simulink model "network_motif_controller_linear_biological_optimisehill"  (R2022b)
settings: Solver=ode4  StartTime=0.0  StopTime=8000-0*5950  FixedStep=0.1  RelTol=1e-3
settings Model: Creator=u1473578  LastModifiedBy=u1473578
settings DebuggingCC: UnconnectedInputMsg=warning  UnconnectedOutputMsg=warning  UnconnectedLineMsg=warning
settings ModelReferenceCC: EnableRefExpFcnMdlSchedulingChecks=on
settings RTWCC: DLArmComputeVersion=19.05

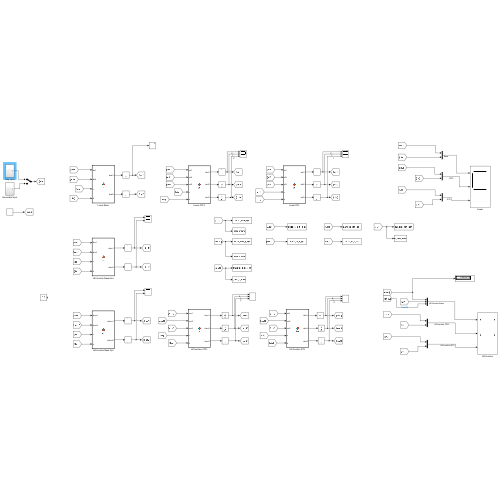
[thumbnail: Simulink's stored preview of the top-level diagram]
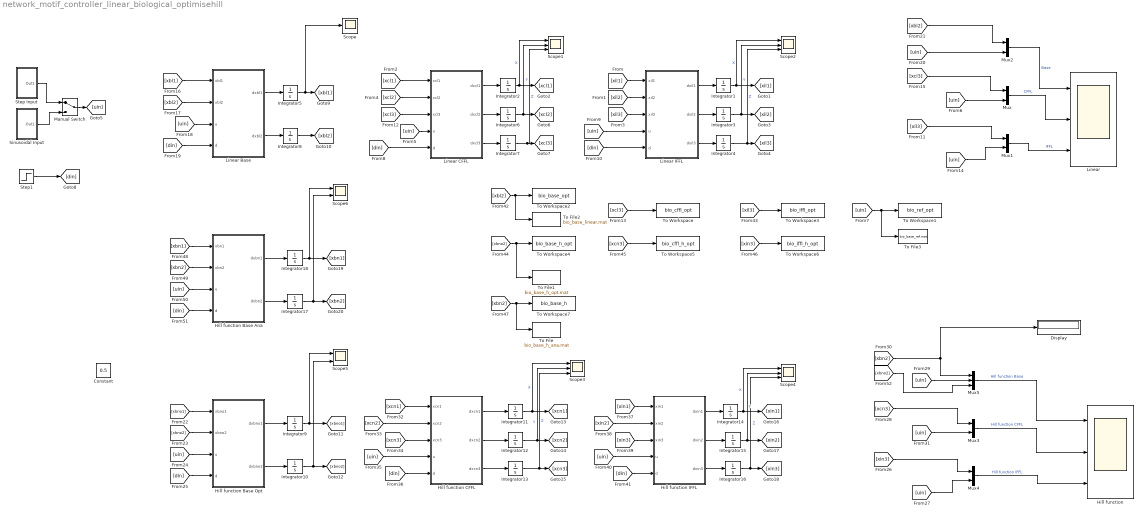
== system network_motif_controller_linear_biological_optimisehill ==
  Constant : Constant  Value=0.5
  Display : Display
  Hill function : Scope  NumInputPorts=3
  Hill function Base Ana : MATLAB Function  TreatAsAtomicUnit=on
  Hill function Base Opt : MATLAB Function  TreatAsAtomicUnit=on
  Hill function CFFL : MATLAB Function  TreatAsAtomicUnit=on
  Hill function IFFL : MATLAB Function  TreatAsAtomicUnit=on
  Integrator{1..18} (18 alike) : Integrator
  Linear : Scope  NumInputPorts=3
  Linear Base : MATLAB Function  TreatAsAtomicUnit=on
  Linear CFFL : MATLAB Function  TreatAsAtomicUnit=on
  Linear IFFL : MATLAB Function  TreatAsAtomicUnit=on
  Manual Switch : ManualSwitch
  Mux{,1..4} (5 alike) : Mux  Inputs=2
  Mux5 : Mux  Inputs=3
  Scope : Scope
  Scope{1..4} (4 alike) : Scope  NumInputPorts=3
  Scope5 : Scope  NumInputPorts=2
  Scope6 : Scope  NumInputPorts=2
  Sinusoidal Input : Subsystem
  Step Input : Subsystem
  Step1 : Step  Time=3000-0*1000  After=1*0.05*(-5e-4)  SampleTime=0
  To File : ToFile  Filename=bio_base_h_ana.mat  MatrixName=xbna2  SaveFormat=Timeseries
  To File1 : ToFile  Filename=bio_base_h_opt.mat  MatrixName=xbno2  SaveFormat=Timeseries
  To File2 : ToFile  Filename=bio_base_linear.mat  MatrixName=xbl2  SaveFormat=Timeseries
  To File3 : ToFile  Filename=bio_base_ref.mat  MatrixName=uref  SaveFormat=Timeseries
  To Workspace : ToWorkspace  VariableName=bio_cffl_opt  SaveFormat=Timeseries  SampleTime=-1
  To Workspace1 : ToWorkspace  VariableName=bio_ref_opt  SaveFormat=Timeseries  SampleTime=-1
  To Workspace2 : ToWorkspace  VariableName=bio_base_opt  SaveFormat=Timeseries  SampleTime=-1
  To Workspace3 : ToWorkspace  VariableName=bio_iffl_opt  SaveFormat=Timeseries  SampleTime=-1
  To Workspace4 : ToWorkspace  VariableName=bio_base_h_opt  SaveFormat=Timeseries  SampleTime=-1
  To Workspace5 : ToWorkspace  VariableName=bio_cffl_h_opt  SaveFormat=Timeseries  SampleTime=-1
  To Workspace6 : ToWorkspace  VariableName=bio_iffl_h_opt  SaveFormat=Timeseries  SampleTime=-1
  To Workspace7 : ToWorkspace  VariableName=bio_base_h  SaveFormat=Timeseries  SampleTime=-1
  wires:
  Integrator2/1 -> Scope1/1, [xcl1]  "X"
  Linear CFFL/3(dxcl3) -> Integrator7/1
  [xcl1] -> Linear CFFL/1(xcl1)
  Integrator7/1 -> Scope1/3, [xcl3]  "Z"
  [xcl2] -> Linear CFFL/2(xcl2)
  [xcl3] -> Linear CFFL/3(xcl3)
  Linear CFFL/2(dxcl2) -> Integrator6/1
  Integrator6/1 -> Scope1/2, [xcl2]  "Y"
  Linear CFFL/1(dxcl1) -> Integrator2/1
  Step Input/1(Out1) -> Manual Switch/1
  Sinusoidal Input/1(Out1) -> Manual Switch/2
  Linear IFFL/1(dxil1) -> Integrator1/1
  Linear IFFL/2(dxil2) -> Integrator3/1
  Linear IFFL/3(dxil3) -> Integrator4/1
  Integrator1/1 -> Scope2/1, [xil1]  "X"
  Integrator3/1 -> Scope2/2, [xil2]  "Y"
  Integrator4/1 -> Scope2/3, [xil3]  "Z"
  [xil1] -> Linear IFFL/1(xil1)
  [xil2] -> Linear IFFL/2(xil2)
  [xil3] -> Linear IFFL/3(xil3)
  Manual Switch/1 -> [uin]
  [uin] -> Linear CFFL/4(u)
  [uin] -> To File3/1, To Workspace1/1
  Step1/1 -> [din]
  [din] -> Linear CFFL/5(d)
  [uin] -> Linear IFFL/4(u)
  [din] -> Linear IFFL/5(d)
  [xcl3] -> To Workspace/1
  Mux/1 -> Linear/2  "CFFL"
  Mux1/1 -> Linear/3  "IFFL"
  [uin] -> Mux/2
  [xcl3] -> Mux/1
  [xil3] -> Mux1/1
  [uin] -> Mux1/2
  Linear Base/1(dxbl1) -> Integrator5/1
  Linear Base/2(dxbl2) -> Integrator8/1
  Integrator5/1 -> Scope/1, [xbl1]
  Integrator8/1 -> [xbl2]
  [xbl1] -> Linear Base/1(xbl1)
  [xbl2] -> Linear Base/2(xbl2)
  [uin] -> Linear Base/3(u)
  [din] -> Linear Base/4(d)
  Mux2/1 -> Linear/1  "Base"
  [xbl2] -> Mux2/1
  [uin] -> Mux2/2
  Hill function Base Opt/1(dxbno1) -> Integrator9/1
  Hill function Base Opt/2(dxbno2) -> Integrator10/1
  Integrator9/1 -> Scope5/1, [xbno1]
  Integrator10/1 -> Scope5/2, [xbno2]
  [xbno1] -> Hill function Base Opt/1(xbno1)
  [xbno2] -> Hill function Base Opt/2(xbno2)
  [din] -> Hill function Base Opt/4(d)
  [xbn2] -> Mux5/1, Display/1
  Mux5/1 -> Hill function/1  "Hill function Base"
  [uin] -> Mux4/2
  [xin3] -> Mux4/1
  [xcn3] -> Mux3/1
  [uin] -> Mux3/2
  Mux4/1 -> Hill function/3  "Hill function IFFL"
  Mux3/1 -> Hill function/2  "Hill function CFFL"
  Hill function CFFL/1(dxcn1) -> Integrator11/1
  Hill function CFFL/2(dxcn2) -> Integrator12/1
  Hill function CFFL/3(dxcn3) -> Integrator13/1
  [xcn1] -> Hill function CFFL/1(xcn1)
  [xcn2] -> Hill function CFFL/2(xcn2)
  [xcn3] -> Hill function CFFL/3(xcn3)
  [uin] -> Hill function CFFL/4(u)
  [din] -> Hill function CFFL/5(d)
  Integrator11/1 -> Scope3/1, [xcn1]  "X"
  Integrator12/1 -> Scope3/2, [xcn2]  "Y"
  Integrator13/1 -> Scope3/3, [xcn3]  "Z"
  Hill function IFFL/1(dxin1) -> Integrator14/1
  Hill function IFFL/2(dxin2) -> Integrator15/1
  Hill function IFFL/3(dxin3) -> Integrator16/1
  Integrator14/1 -> Scope4/1, [xin1]  "X"
  Integrator15/1 -> Scope4/2, [xin2]  "Y"
  Integrator16/1 -> Scope4/3, [xin3]  "Z"
  [xin1] -> Hill function IFFL/1(xin1)
  [xin2] -> Hill function IFFL/2(xin2)
  [xin3] -> Hill function IFFL/3(xin3)
  [uin] -> Hill function IFFL/4(u)
  [din] -> Hill function IFFL/5(d)
  [xbl2] -> To File2/1, To Workspace2/1
  [xil3] -> To Workspace3/1
  [uin] -> Hill function Base Opt/3(u)
  [xbno2] -> To File1/1, To Workspace4/1
  [xcn3] -> To Workspace5/1
  [xin3] -> To Workspace6/1
  [xbn2] -> To File/1, To Workspace7/1
  Hill function Base Ana/1(dxbn1) -> Integrator18/1
  [din] -> Hill function Base Ana/4(d)
  [xbn2] -> Hill function Base Ana/2(xbn2)
  Integrator17/1 -> Scope6/2, [xbn2]
  [uin] -> Hill function Base Ana/3(u)
  [xbn1] -> Hill function Base Ana/1(xbn1)
  Integrator18/1 -> Scope6/1, [xbn1]
  Hill function Base Ana/2(dxbn2) -> Integrator17/1
  [uin] -> Mux5/2
  [xbno2] -> Mux5/3

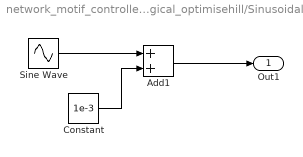
== system network_motif_controller_linear_biological_optimisehill/Sinusoidal Input ==
  Add1 : Sum
  Constant : Constant  Value=1e-3
  Sine Wave : Sin  Amplitude=1e-3  Frequency=10/6000  Phase=2800-150  SampleTime=0
  Out1 : Outport
  wires:
  Sine Wave/1 -> Add1/1
  Constant/1 -> Add1/2
  Add1/1 -> Out1/1

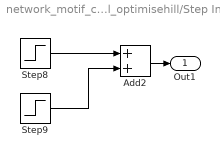
== system network_motif_controller_linear_biological_optimisehill/Step Input ==
  Add2 : Sum
  Step8 : Step  Time=0  After=0  SampleTime=0
  Step9 : Step  Time=1000  After=1e-3  SampleTime=0
  Out1 : Outport
  wires:
  Step9/1 -> Add2/2
  Step8/1 -> Add2/1
  Add2/1 -> Out1/1

== matlab function network_motif_controller_linear_biological_optimisehill/Linear IFFL ==
  data: xil1 input; xil2 input; xil3 input; u input; dxil1 output; dxil2 output; d input; dxil3 output
function [dxil1,dxil2,dxil3] = fcn(xil1,xil2,xil3,u,d)

% x1 = X
% x2 = Y
% x3 = Z

gamma = 1;
c = gamma;
% % per second
% delta_x = 0.001;
% delta_y = 0.004;
% delta_z = 0.004;

% per minutes
delta_x = 0.0005;
delta_y = 0.02;
delta_z = 0.02;

% % per hour
% delta_x = 0.0013;
% delta_y = 0.1;
% delta_z = 0.1;

alpha_y = 0.0005;
alpha_z1 = 0.0005;
alpha_z2 = 0.0005;



dxil1 = c*u - gamma*xil3 - delta_x*xil1;

dxil2 = alpha_y*xil1 - delta_y*xil2;

dxil3 = alpha_z1*xil1 - alpha_z2*xil2 - delta_z*xil3 + 1*d;

== matlab function network_motif_controller_linear_biological_optimisehill/Linear Base ==
  data: xbl1 input; xbl2 input; u input; dxbl1 output; dxbl2 output; d input
function [dxbl1,dxbl2] = fcn(xbl1,xbl2,u,d)

% x1 = X
% x2 = Z

gamma = 1;
c = gamma;

% % per second
% delta_x = 0.001;
% delta_y = 0.004;
% delta_z = 0.004;

% per minutes
delta_x = 0.0005;
delta_z = 0.02;

% % per hour
% delta_x = 0.0013;
% delta_y = 0.1;
% delta_z = 0.1;

alpha_z = 0.0005;


bs = 0*5e-3;

dxbl1 = c*u - gamma*xbl2 - delta_x*xbl1 + bs;

dxbl2 = alpha_z*xbl1 - delta_z*xbl2 + 1*d;

== matlab function network_motif_controller_linear_biological_optimisehill/Hill function Base Opt ==
  data: xbno1 input; xbno2 input; u input; dxbno1 output; dxbno2 output; d input
function [dxbno1,dxbno2] = fcn(xbno1,xbno2,u,d)

% x1 = X
% x2 = Z

gamma = 1;
c = gamma;
%% Derived Parameters through two-point matching (Inhibition Type 1)
% Kx = 0.002;
% Kz = 0.08;
% 
% % per minutes
% delta_x = 0.0005;
% delta_z = 0.02;
% 
% alpha_x = 2e-8;
% alpha_z = 1e-4;
% 
% bs = -5e-3;

%% Derived Parameters through two-point matching (Inhibition Type 2)
% Kx = 0.002; % analytic
Kx = 0.0022; % optimise
% Kz = 0.08; % analytic
Kz = 0.1896; % optimise

% per minutes
delta_x = 0.0005;
delta_z = 0.02;

% alpha_x = 0.005; % analytic
alpha_x = 0.0051; % optimise
% alpha_z = 1e-4; % analytic
alpha_z = 2e-4; % optimise

bs = -5e-3;


%% Matthew's Parameters (Inhibiition Type 2)
% Kx = sqrt(0.05);
% Kz = sqrt(0.05);
% 
% % per minutes
% delta_x = 0.5;
% delta_z = 0.5;
% 
% alpha_x = 0.5;
% alpha_z = 0.5;
% 
% bs = -0.5;

%% ODE

% Inhibition Type 1
% dxbn1 = c*u + ((alpha_x)/(Kx^2 + xbn2^2) + bs) - delta_x*xbn1;

% Inhibition Type 2
dxbno1 = c*u + ((alpha_x*Kx^2)/(Kx^2 + xbno2^2) + bs) - delta_x*xbno1;

dxbno2 = (alpha_z*xbno1^2/(Kz^2 + xbno1^2)) - delta_z*xbno2 + 1*d;

== matlab function network_motif_controller_linear_biological_optimisehill/Linear CFFL ==
  data: xcl1 input; xcl2 input; xcl3 input; u input; dxcl1 output; dxcl2 output; d input; dxcl3 output
function [dxcl1,dxcl2,dxcl3] = fcn(xcl1,xcl2,xcl3,u,d)

% x1 = X
% x2 = Y
% x3 = Z

gamma = 1;
c =  gamma;
% % per second
% delta_x = 0.001;
% delta_y = 0.004;
% delta_z = 0.004;

% per minutes
delta_x = 0.0005;
delta_y = 0.02;
delta_z = 0.02;

% % per hour
% delta_x = 0.0013;
% delta_y = 0.1;
% delta_z = 0.1;

alpha_y = 0.0005;
alpha_z1 = 0.0005;
alpha_z2 = 0.0005;



dxcl1 = c*u - gamma*xcl3 - delta_x*xcl1;

dxcl2 = alpha_y*xcl1 - delta_y*xcl2;

dxcl3 = alpha_z1*xcl1 + alpha_z2*xcl2 - delta_z*xcl3 + 1*d;

== matlab function network_motif_controller_linear_biological_optimisehill/Hill function CFFL ==
  data: xcn1 input; xcn2 input; xcn3 input; u input; dxcn1 output; dxcn2 output; d input; dxcn3 output
function [dxcn1,dxcn2,dxcn3] = fcn(xcn1,xcn2,xcn3,u,d)

% x1 = X
% x2 = Z

gamma = 1;
c = gamma;
%% Derived Parameters through two-point matching (Inhibition Type 1)
% Kx = 0.002;
% Kz = 0.08;
% 
% % per minutes
% delta_x = 0.0005;
% delta_z = 0.02;
% 
% alpha_x = 2e-8;
% alpha_z = 1e-4;
% 
% bs = -5e-3;

%% Derived Parameters through two-point matching (Inhibition Type 2)
Kx = 0.002;
Ky = 0.08; 
Kz1 = 0.08; 
% Kz2 = 0.08; 
Kz2 = 0.001385467691241;

% per minutes
delta_x = 0.0005;
delta_y = 0.02;
delta_z = 0.02;

alpha_x = 0.005;
alpha_y = 0.0001; 
alpha_z1 = 0.0001; 
% alpha_z2 = 0.0001; 
alpha_z2 = 0.000002149155370;

bs = -0.005;


%% Matthew's Parameters (Inhibiition Type 2)
% Kx = 0.05;
% Kz = 0.05;
% 
% % per minutes
% delta_x = 0.5;
% delta_z = 0.5;
% 
% alpha_x = 0.5;
% alpha_z = 0.5;
% 
% bs = -0.5;

%% ODE

% Inhibition Type 1
% dxbn1 = c*u + ((alpha_x)/(Kx^2 + xbn2^2) + bs) - delta_x*xbn1;

% Inhibition Type 2
dxcn1 = c*u + ((alpha_x*Kx^2)/(Kx^2 + xcn3^2) + bs) - delta_x*xcn1;

dxcn2 = (alpha_y*xcn1^2)/(Ky^2 + xcn1^2) - delta_y*xcn2;

dxcn3 = (alpha_z1*xcn1^2/(Kz1^2 + xcn1^2)) + (alpha_z2*xcn2^2/(Kz2^2 + xcn2^2)) - delta_z*xcn3 + 1*d;

== matlab function network_motif_controller_linear_biological_optimisehill/Hill function IFFL ==
  data: xin1 input; xin2 input; xin3 input; u input; dxin1 output; dxin2 output; d input; dxin3 output
function [dxin1,dxin2,dxin3] = fcn(xin1,xin2,xin3,u,d)

% x1 = X
% x2 = Z

gamma = 1;
c = gamma;
%% Derived Parameters through two-point matching (Inhibition Type 1)
% Kx = 0.002;
% Kz = 0.08;
% 
% % per minutes
% delta_x = 0.0005;
% delta_z = 0.02;
% 
% alpha_x = 2e-8;
% alpha_z = 1e-4;
% 
% bs = -5e-3;

%% Derived Parameters through two-point matching (Inhibition Type 2)
Kx = 0.002;
Ky = 0.08; 

% % 2-Term
Kz1 = 0.08;
Kz2 = 0.2683;

% % 4DOF
% Kz1 = 0.6599; 
% Kz2 = 0.3168; 

% 2DOF
Kz = 0.1497;

% per minutes
delta_x = 0.0005;
delta_y = 0.02;
delta_z = 0.02;

alpha_x = 0.005;
alpha_y = 0.0001; 

% % 2-Term
alpha_z1 = 1e-4;
alpha_z2 = 0.006;

% % 4DOF
% alpha_z1 = 0.0022; 
% alpha_z2 = 0.8398; 

% 2DOF
alpha_z = 0.0027;

bs = -0.005;
bsz = -0.006;

%% Matthew's Parameters (Inhibiition Type 2)
% Kx = 0.05;
% Kz = 0.05;
% 
% % per minutes
% delta_x = 0.5;
% delta_z = 0.5;
% 
% alpha_x = 0.5;
% alpha_z = 0.5;
% 
% bs = -0.5;

%% ODE

% Inhibition Type 1
% dxbn1 = c*u + ((alpha_x)/(Kx^2 + xbn2^2) + bs) - delta_x*xbn1;

% Inhibition Type 2
dxin1 = c*u + ((alpha_x*Kx^2)/(Kx^2 + xin3^2) + bs) - delta_x*xin1;

dxin2 = (alpha_y*xin1^2)/(Ky^2 + xin1^2) - delta_y*xin2;

dxin3 = (alpha_z1*xin1^2/(Kz1^2 + xin1^2)) + (alpha_z2*Kz2^2/(Kz2^2 + xin2^2) + bsz) - delta_z*xin3 + 1*d; % 2-term
% dxin3 = (alpha_z1*alpha_z2*Kz2^2*xin1^2)/((Kz1^2 + xin1^2)*(Kz2^2 + xin1^2)) - delta_z*xin3 + 1*d; % 4DOF
% dxin3 = (alpha_z^2*xin1^2)/((Kz^2 + xin1^2)*(Kz^2 + xin1^2)) - delta_z*xin3 + 1*d; % 2DOF

== matlab function network_motif_controller_linear_biological_optimisehill/Hill function Base Ana ==
  data: xbn1 input; xbn2 input; u input; dxbn1 output; dxbn2 output; d input
function [dxbn1,dxbn2] = fcn(xbn1,xbn2,u,d)

% x1 = X
% x2 = Z

gamma = 1;
c = gamma;
%% Derived Parameters through two-point matching (Inhibition Type 1)
% Kx = 0.002;
% Kz = 0.08;
% 
% % per minutes
% delta_x = 0.0005;
% delta_z = 0.02;
% 
% alpha_x = 2e-8;
% alpha_z = 1e-4;
% 
% bs = -5e-3;

%% Derived Parameters through two-point matching (Inhibition Type 2)
Kx = 0.002;
Kz = 0.08;

% per minutes
delta_x = 0.0005;
delta_z = 0.02;

alpha_x = 0.005;
alpha_z = 1e-4;

bs = -5e-3;


%% Matthew's Parameters (Inhibiition Type 2)
% Kx = sqrt(0.05);
% Kz = sqrt(0.05);
% 
% % per minutes
% delta_x = 0.5;
% delta_z = 0.5;
% 
% alpha_x = 0.5;
% alpha_z = 0.5;
% 
% bs = -0.5;

%% ODE

% Inhibition Type 1
% dxbn1 = c*u + ((alpha_x)/(Kx^2 + xbn2^2) + bs) - delta_x*xbn1;

% Inhibition Type 2
dxbn1 = c*u + ((alpha_x*Kx^2)/(Kx^2 + xbn2^2) + bs) - delta_x*xbn1;

dxbn2 = (alpha_z*xbn1^2/(Kz^2 + xbn1^2)) - delta_z*xbn2 + 1*d;
